simulink model "intro_1"  (R2025b)
settings: Solver=FixedStepAuto  StartTime=0.0  StopTime=10.0  FixedStep=1e-4  RelTol=1e-3
values from neighbouring files (symbols this model uses):
  a = 0.2    [setup.m]
  omega = 5    [setup.m]
  qbar = 1.5    [setup.m]
settings Model: Creator=seby  LastModifiedBy=seby

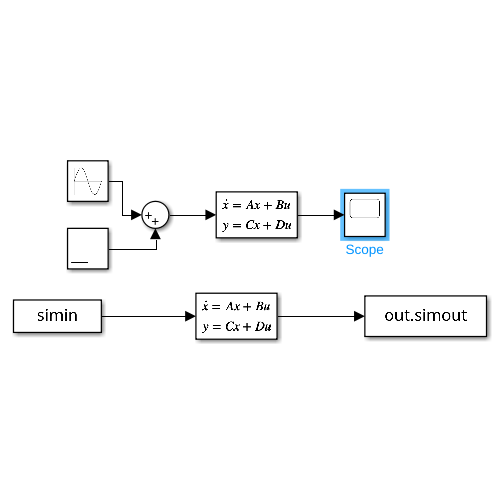
[thumbnail: Simulink's stored preview of the top-level diagram]
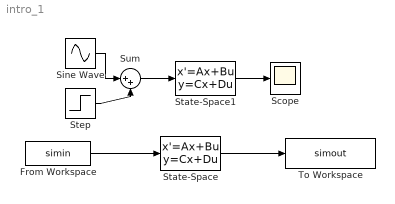
== system intro_1 ==
  From Workspace : FromWorkspace  VariableName=simin
  Scope : Scope
      settings: ActiveDisplayYMinimum=0.33861255680229796  ActiveDisplayYMaximum=1.7098882568884859
  Sine Wave : Sin  Amplitude=a  Frequency=omega  SampleTime=0
  State-Space : StateSpace  A=[-3 0; 3 -5]  B=[1;0]  C=[0 5]  D=[0]  InitialCondition=[0.1;0.1]
  State-Space1 : StateSpace  A=[-3 0; 3 -5]  B=[1;0]  C=[0 5]  D=[0]  InitialCondition=[0.1;0.1]
  Step : Step  Time=0  After=qbar  SampleTime=0
  Sum : Sum  Inputs=|++
  To Workspace : ToWorkspace  VariableName=simout  SaveFormat=Timeseries  SampleTime=-1
  wires:
  From Workspace/1 -> State-Space/1
  State-Space/1 -> To Workspace/1
  Step/1 -> Sum/2
  Sine Wave/1 -> Sum/1
  State-Space1/1 -> Scope/1
  Sum/1 -> State-Space1/1
